simulink model "simpleMassSipringDamperModel"  (R2020b)
settings: Solver=FixedStepAuto  StartTime=0.0  StopTime=10.0  FixedStep=1e-3  RelTol=1e-3
settings Model: Creator=kuzub  LastModifiedBy=kuzub

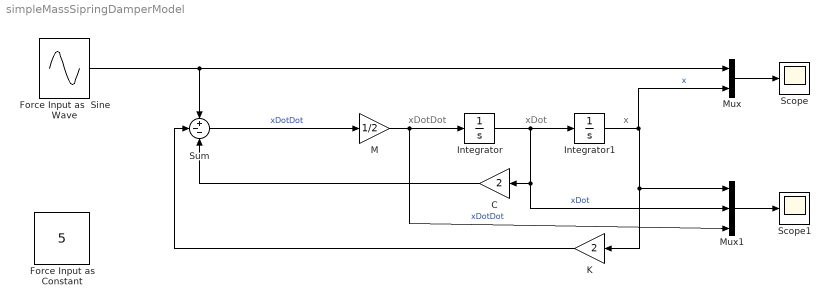
== system simpleMassSipringDamperModel ==
  note: xDotDot
  note: xDot
  note: x
  C : Gain  Gain=2
  Force Input as  Sine Wave : Sin  Amplitude=5  Bias=5  Frequency=2*pi*1  SampleTime=0
  Force Input as Constant : Constant  Value=5
  Integrator : Integrator
  Integrator1 : Integrator
  K : Gain  Gain=2
  M : Gain  Gain=1/2
  Mux : Mux  Inputs=2
  Mux1 : Mux  Inputs=3
  Scope : Scope
  Scope1 : Scope
  Sum : Sum  Inputs=+--
  wires:
  Mux1/1 -> Scope1/1
  K/1 -> Sum/2
  C/1 -> Sum/3
  Force Input as  Sine Wave/1 -> Mux/1, Sum/1
  Integrator/1 -> Mux1/2, C/1, Integrator1/1  "xDot"
  M/1 -> Mux1/3, Integrator/1  "xDotDot"
  Mux/1 -> Scope/1
  Sum/1 -> M/1  "xDotDot"
  Integrator1/1 -> Mux/2, K/1, Mux1/1  "x"
